simulink model "Sim_Model"  (R2021a)
settings: Solver=VariableStepAuto  StartTime=0.0  StopTime=10  RelTol=1e-3
libraries: simulink x2
settings Model: Creator=hmahmood  LastModifiedBy=ryans
settings SolverCC: AlgebraicLoopSolver=TrustRegion
settings DebuggingCC: SFMachineParentedDataDiag=warning

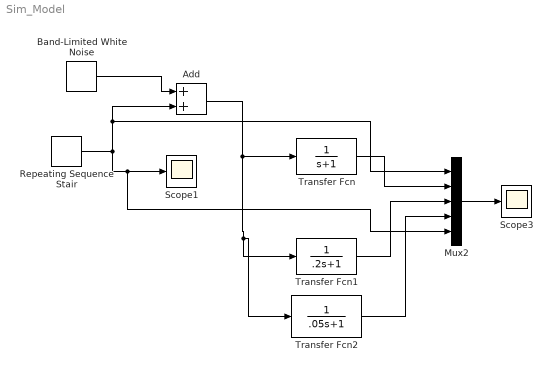
== system Sim_Model ==
  Add : Sum
  Band-Limited White Noise : simulink/Sources/Band-Limited White Noise  Cov=[0.00001]  Ts=0.004  seed=[23341]
  Mux2 : Mux  Inputs=5
  Repeating Sequence Stair : simulink/Sources/Repeating Sequence Stair  OutValues=[2 2.25 2.5 2.6 2.7].'  tsamp=2  OutMin=[]  OutMax=[]  OutDataTypeStr=double  OutputDataTypeScalingMode=double  OutDataType=fixdt(0,8)  ConRadixGroup=Best Precision: Vector-wise  OutScaling=2^-12
  Scope1 : Scope
  Scope3 : Scope
  Transfer Fcn : TransferFcn  Denominator=[1 1]
  Transfer Fcn1 : TransferFcn  Denominator=[.2 1]
  Transfer Fcn2 : TransferFcn  Denominator=[.05 1]
  wires:
  Repeating Sequence Stair/1 -> Mux2/1, Add/2, Mux2/5, Scope1/1
  Transfer Fcn1/1 -> Mux2/3
  Add/1 -> Transfer Fcn1/1, Transfer Fcn2/1, Transfer Fcn/1
  Mux2/1 -> Scope3/1
  Transfer Fcn2/1 -> Mux2/4
  Transfer Fcn/1 -> Mux2/2
  Band-Limited White Noise/1 -> Add/1
